simulink model "AC"  (R2020b)
settings: Solver=ode23s  StartTime=0.0  StopTime=9.6  RelTol=1e-3
undefined symbols (not defined in the file): Capacitor, Run, Start
libraries: powerlib x21, powerlib_meascontrol x4
settings Model: Creator=pvdk1  LastModifiedBy=pvdk1

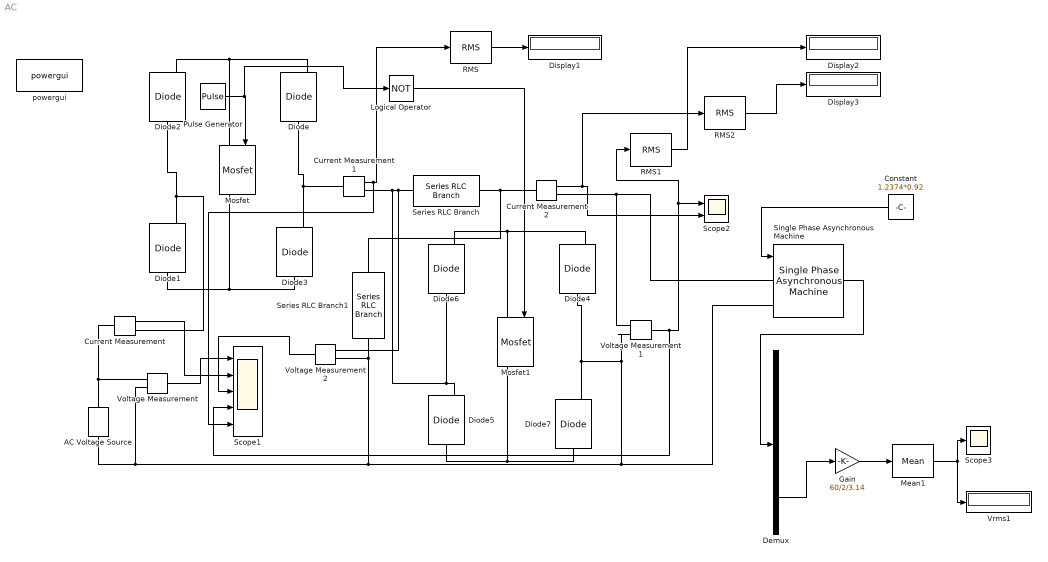
== system AC ==
  AC Voltage Source : powerlib/Electrical Sources/AC Voltage Source  Amplitude=140*sqrt(2)  Phase=0  Frequency=50  SampleTime=0  Measurements=None  BusType=swing  Pref=10e3  Qref=0  Qmin=-inf  Qmax=+inf
  Constant : Constant  Value=1.2374*0.92
  Current Measurement : powerlib/Measurements/Current Measurement  PhasorSimulation=off  OutputType=Complex  PSBequivalent=0
  Current Measurement1 : powerlib/Measurements/Current Measurement  PhasorSimulation=off  OutputType=Complex  PSBequivalent=0
  Current Measurement2 : powerlib/Measurements/Current Measurement  PhasorSimulation=off  OutputType=Complex  PSBequivalent=0
  Demux : Demux  Outputs=14
  Diode{,1..7} (8 alike) : powerlib/Power Electronics/Diode  Ron=0.001  Lon=0  Vf=0.8  IC=0  UseSnubber=0  Rs=5000  Cs=250e-9  Measurements=on
  Display1 : Display
  Display2 : Display
  Display3 : Display
  Gain : Gain  Gain=60/2/3.14
  Logical Operator : Logic  Operator=NOT  AllPortsSameDT=off  OutDataTypeStr=boolean
  Mean1 : powerlib_meascontrol/Measurements/Mean  Freq=50  Vinit=0  Ts=0
  Mosfet : powerlib/Power Electronics/Mosfet  Ron=0.1  Lon=0  Rd=0.01  Vfd=0  IC=0  Rs=5000  Cs=250e-9  Measurements=on
  Mosfet1 : powerlib/Power Electronics/Mosfet  Ron=0.1  Lon=0  Rd=0.01  Vfd=0  IC=0  Rs=5000  Cs=250e-9  Measurements=on
  Pulse Generator : DiscretePulseGenerator  PulseType=Time based  Period=1/1100  PulseWidth=90
  RMS : powerlib_meascontrol/Measurements/RMS  TrueRMS=on  Freq=60  RMSInit=120  Ts=0
  RMS1 : powerlib_meascontrol/Measurements/RMS  TrueRMS=on  Freq=60  RMSInit=120  Ts=0
  RMS2 : powerlib_meascontrol/Measurements/RMS  TrueRMS=on  Freq=60  RMSInit=120  Ts=0
  Scope1 : Scope  NumInputPorts=5
  Scope2 : Scope  NumInputPorts=2
  Scope3 : Scope
  Series RLC Branch : powerlib/Elements/Series RLC Branch  LConnTagsString=__new0  RConnTagsString=__new0  BranchType=RL  Resistance=0.2  Inductance=5e-3  SetiL0=off  InitialCurrent=0  Capacitance=1e-6  Setx0=off  InitialVoltage=0  Measurements=None
  Series RLC Branch1 : powerlib/Elements/Series RLC Branch  LConnTagsString=__new0  RConnTagsString=__new0  BranchType=RC  Resistance=0.1  Inductance=1e-3  SetiL0=off  InitialCurrent=0  Capacitance=63e-6  Setx0=off  InitialVoltage=0  Measurements=None
  Single Phase Asynchronous Machine : powerlib/Machines/Single Phase Asynchronous Machine  MechanicalLoad=Torque Tm  UNITS=SI  MachineType=Capacitor-Start-Run  MeasurementBus=off  NominalParameters="[ .25*746  110  50]"  MainWindingStator="[2.02  7.4e-3]"  MainWindingRotor="[4.12  5.6e-3]"  MutualInductance=0.1772  AuxiliaryWinding="[7.14  8.5e-3]"  Mechanical="[0.0146  0  2 1.18]"  CapacitorStart="[2  254.7e-6]"  CapacitorRun="[18  21.1e-6]"  DisconnectionSpeed=75  InitialSpeed=0  DataType=SI  TsPowergui=0  TsBlock=-1
      settings: SourceProductBaseCode=PS
  Voltage Measurement : powerlib/Measurements/Voltage Measurement  PhasorSimulation=off  OutputType=Complex  PSBequivalent=0
  Voltage Measurement1 : powerlib/Measurements/Voltage Measurement  PhasorSimulation=off  OutputType=Complex  PSBequivalent=0
  Voltage Measurement2 : powerlib/Measurements/Voltage Measurement  PhasorSimulation=off  OutputType=Complex  PSBequivalent=0
  Vrms1 : Display
  powergui : powerlib/powergui  Priority=1  SimulationMode=Continuous  SampleTime=50e-6  frequency=60  Iterations=50  frequencyindice=50  Pbase=100e6  ErrMax=1e-4  UnitsV=kV  UnitsW=MW  buscounter=0  FunctionMessages=off  echomessages=off  EnableUseOfTLC=off  CurrentSourceSwitches=off  DisableSnubberDevices=off  DisableRonSwitches=off  DisableVfSwitches=off  DisplayEquations=off  AutomaticDiscreteSolvers=off  SolverType=Tustin/Backward Euler (TBE)  Interpol=off  ExternalGateDelay=off  methode=off  Ts=100  x0status=blocks  SPID=on  SwTol=0  HookPort=off  NonlinearTolerance=1e-4  nMaxIteration=100  ContinueOnMaxIteration=off  RestoreLinks=warning  ResistiveCurrentMeasurement=off  Frange=[0:2:500]  Ylog=off  Xlog=on  ShowGrid=off  save=off  variable=ZData  structure=0  ZoomFFT=off  StartTime=0.0  cycles=1  DisplayStyle=1  fundamental=60  FreqAxis=off  MaxFrequency=1000  frequencyindicesteady=1  RmsSteady=1  display=off
  wires:
  Pulse Generator/1 -> Logical Operator/1, Mosfet/1
  Current Measurement1/1 -> Scope1/5, RMS/1
  RMS/1 -> Display1/1
  Logical Operator/1 -> Mosfet1/1
  Current Measurement/1 -> Scope1/2
  Voltage Measurement/1 -> Scope1/1
  RMS2/1 -> Display3/1
  RMS1/1 -> Display2/1
  Voltage Measurement1/1 -> Scope1/4, RMS1/1, Scope2/1
  Current Measurement2/1 -> RMS2/1, Scope2/2
  Single Phase Asynchronous Machine/1 -> Demux/1
  Gain/1 -> Mean1/1
  Mean1/1 -> Vrms1/1, Scope3/1
  Demux/12 -> Gain/1
  Constant/1 -> Single Phase Asynchronous Machine/1
  Voltage Measurement2/1 -> Scope1/3
  connections:
  AC Voltage Source/RConn1 -- Voltage Measurement/LConn1 -- Current Measurement/LConn1
  Voltage Measurement/LConn2 -- Voltage Measurement2/LConn1 -- Series RLC Branch1/RConn1 -- Diode7/RConn1 -- Diode4/LConn1 -- Voltage Measurement1/LConn2 -- Single Phase Asynchronous Machine/LConn2 -- AC Voltage Source/LConn1
  Diode2/LConn1 -- Current Measurement/RConn1 -- Diode1/RConn1
  Diode1/LConn1 -- Mosfet/RConn1 -- Diode3/LConn1
  Diode3/RConn1 -- Current Measurement1/LConn1 -- Diode/LConn1
  Diode2/RConn1 -- Mosfet/LConn1 -- Diode/RConn1
  Series RLC Branch/LConn1 -- Current Measurement1/RConn1 -- Diode5/RConn1 -- Diode6/LConn1 -- Voltage Measurement2/LConn2
  Diode6/RConn1 -- Mosfet1/LConn1 -- Diode4/RConn1
  Diode5/LConn1 -- Mosfet1/RConn1 -- Diode7/LConn1
  Series RLC Branch/RConn1 -- Series RLC Branch1/LConn1 -- Current Measurement2/LConn1
  Current Measurement2/RConn1 -- Voltage Measurement1/LConn1 -- Single Phase Asynchronous Machine/LConn1
